simulink model "model a"  (R2023b)
settings: Solver=VariableStepAuto  StartTime=0.0  StopTime=10.0  RelTol=1e-3
settings Model: Creator=R.Dipti  LastModifiedBy=R.Dipti

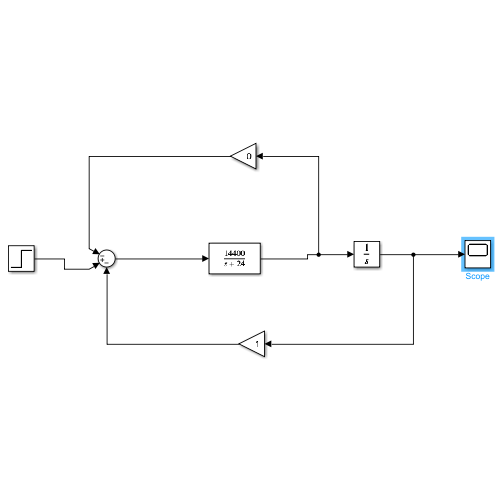
[thumbnail: Simulink's stored preview of the top-level diagram]
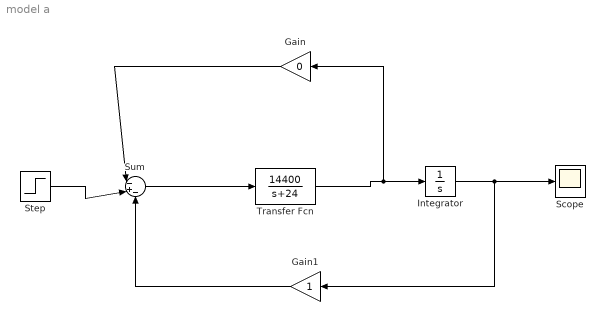
== system model a ==
  Gain : Gain  Gain=0
  Gain1 : Gain
  Integrator : Integrator
  Scope : Scope
  Step : Step  SampleTime=0
  Sum : Sum  Inputs=|-+-
  Transfer Fcn : TransferFcn  Numerator=[14400]  Denominator=[1 24]
  wires:
  Step/1 -> Sum/2
  Gain/1 -> Sum/1
  Gain1/1 -> Sum/3
  Sum/1 -> Transfer Fcn/1
  Transfer Fcn/1 -> Gain/1, Integrator/1
  Integrator/1 -> Gain1/1, Scope/1
